simulink model "TEST_MaskRadioButtons_model"  (R2018b)
settings: Solver=VariableStepAuto  StartTime=0.0  StopTime=10.0  RelTol=1e-3
libraries: MaskRadioButtons_library x2
settings Model: Creator=Christopher  LastModifiedBy=Christopher

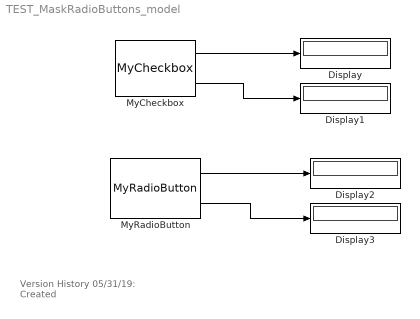
== system TEST_MaskRadioButtons_model ==
  note: Version History
      | 05/31/19: Created
  Display{,1..3} (4 alike) : Display
  MyCheckbox : MaskRadioButtons_library/MyCheckbox  cruiseControl=on  windshieldWipers=on
  MyRadioButton : MaskRadioButtons_library/MyRadioButton  vehicle=Car  engineSystem=Squirrel
  wires:
  MyCheckbox/1 -> Display/1
  MyCheckbox/2 -> Display1/1
  MyRadioButton/1 -> Display2/1
  MyRadioButton/2 -> Display3/1
